simulink model "LAB6ADAsim"  (R2024a)
settings: Solver=VariableStepAuto  StartTime=0.0  StopTime=10.0  RelTol=1e-3
libraries: cstblocks x2
settings Model: Creator=alifuatsakaci  LastModifiedBy=alifuatsakaci

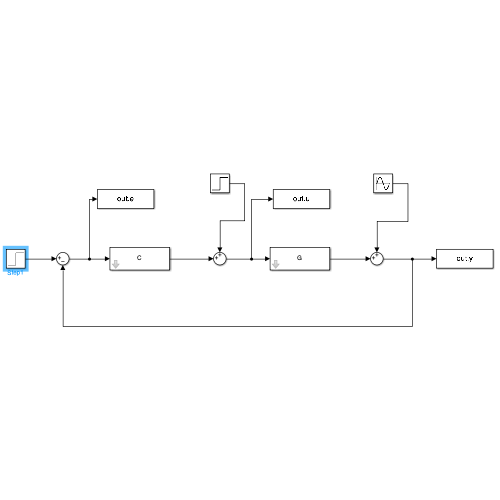
[thumbnail: Simulink's stored preview of the top-level diagram]
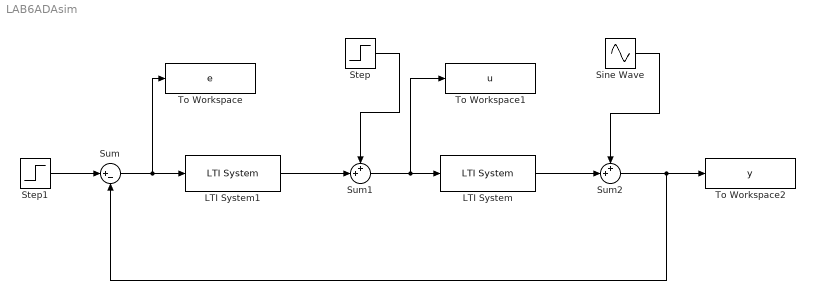
== system LAB6ADAsim ==
  LTI System : cstblocks/LTI System  sys=G  IC=[]  PadeOrder=0
  LTI System1 : cstblocks/LTI System  sys=C  IC=[]  PadeOrder=0
  Sine Wave : Sin  Amplitude=0  Frequency=0  SampleTime=0
  Step : Step  Time=0  After=0  SampleTime=0
  Step1 : Step  Time=0  SampleTime=0
  Sum : Sum  Inputs=|+-
  Sum1 : Sum  Inputs=++|
  Sum2 : Sum  Inputs=++|
  To Workspace : ToWorkspace  VariableName=e  SaveFormat=Timeseries  SampleTime=-1
  To Workspace1 : ToWorkspace  VariableName=u  SaveFormat=Timeseries  SampleTime=-1
  To Workspace2 : ToWorkspace  VariableName=y  SaveFormat=Timeseries  SampleTime=-1
  wires:
  Step1/1 -> Sum/1
  Sum/1 -> To Workspace/1, LTI System1/1
  LTI System1/1 -> Sum1/2
  Sum1/1 -> To Workspace1/1, LTI System/1
  Step/1 -> Sum1/1
  Sum2/1 -> Sum/2, To Workspace2/1
  Sine Wave/1 -> Sum2/1
  LTI System/1 -> Sum2/2
